simulink model "blocos"  (R2018a)
settings: Solver=VariableStepAuto  StartTime=0.0  StopTime=10.0  RelTol=1e-3
libraries: dspsnks4 x2
settings Model: Creator=joaovitor  LastModifiedBy=joaovitor

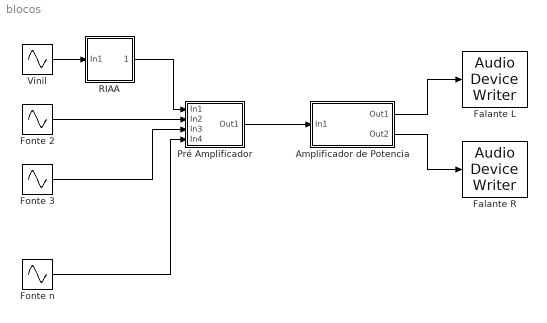
== system blocos ==
  Amplificador de Potencia : Subsystem
  Falante L : dspsnks4/Audio Device Writer  Driver=CoreAudio  Device=Default  InheritSampleRate=on  SampleRate=44100  BitDepth=16-bit integer  BufferSize=4096  NumBuffers=10  DefaultOutputChannelMapping=on  OutputChannelMapping=1:2  OutputNumUnderrunSamples=off  DriverIdx=5  DeviceWarnFlag=''
  Falante R : dspsnks4/Audio Device Writer  Driver=CoreAudio  Device=Default  InheritSampleRate=on  SampleRate=44100  BitDepth=16-bit integer  BufferSize=4096  NumBuffers=10  DefaultOutputChannelMapping=on  OutputChannelMapping=1:2  OutputNumUnderrunSamples=off  DriverIdx=5  DeviceWarnFlag=''
  Fonte 2 : Sin  SampleTime=0
  Fonte 3 : Sin  SampleTime=0
  Fonte n : Sin  SampleTime=0
  Pré Amplificador : Subsystem
  RIAA : Subsystem
  "Vinil " : Sin  SampleTime=0
  wires:
  "Vinil "/1 -> RIAA/1(In1)
  Fonte 2/1 -> Pré Amplificador/2(In2)
  Fonte 3/1 -> Pré Amplificador/3(In3)
  RIAA/1(Out1) -> Pré Amplificador/1(In1)
  Pré Amplificador/1(Out1) -> Amplificador de Potencia/1(In1)
  Amplificador de Potencia/1(Out1) -> Falante L/1
  Fonte n/1 -> Pré Amplificador/4(In4)
  Amplificador de Potencia/2(Out2) -> Falante R/1

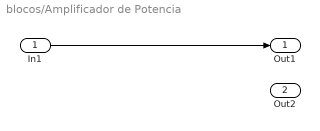
== system blocos/Amplificador de Potencia ==
  In1 : Inport
  Out1 : Outport
  Out2 : Outport  Port=2
  wires:
  In1/1 -> Out1/1

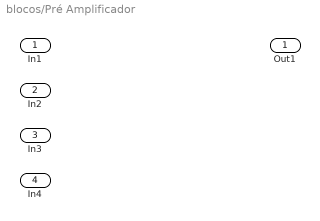
== system blocos/Pré Amplificador ==
  In1 : Inport
  In2 : Inport  Port=2
  In3 : Inport  Port=3
  In4 : Inport  Port=4
  Out1 : Outport

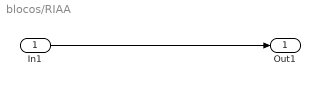
== system blocos/RIAA ==
  In1 : Inport
  Out1 : Outport
  wires:
  In1/1 -> Out1/1
